simulink model "time_gongji_KVHonline"  (R2019b)
settings: Solver=ode3  StartTime=0.0  StopTime=6000  FixedStep=0.01  MaxStep=0.01  RelTol=1e-3
values from neighbouring files (symbols this model uses):
  bias_gyro_z_gongji = 2e-3    (= 0.002)    [sych_ite_KVHonline_daoyuan_huace.m]
settings Model: Creator=luyishi_E480  LastModifiedBy=xie_z
settings DataIOCC: SaveOutput=off  SignalLogging=off  DSMLogging=off  InspectSignalLogs=on  SaveTime=off  ReturnWorkspaceOutputs=off
settings DebuggingCC: InheritedTsInSrcMsg=none

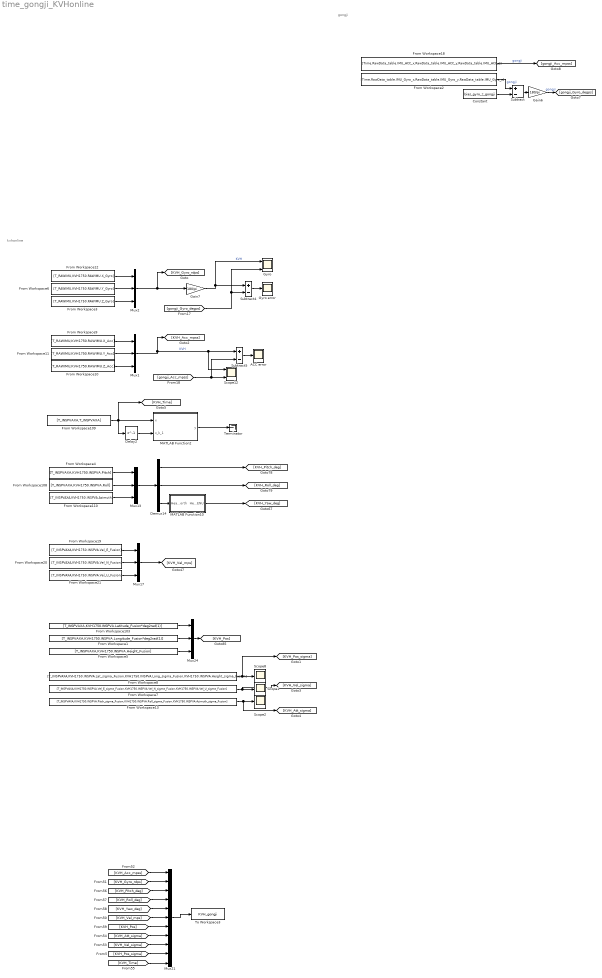
== system time_gongji_KVHonline ==
  note: gongji
  note: kvhonline
  ACC error : Scope
  Constant : Constant  Value=bias_gyro_z_gongji
  Delay2 : Delay  DelayLength=1  InitialCondition=0
  Demux14 : Demux  Outputs=3
  From Workspace1 : FromWorkspace  VariableName=[T_INSPVAXA,KVH1750.INSPVA.Longitude_Fusion*deg2rad(1)]  OutputAfterFinalValue=Holding final value
  From Workspace10 : FromWorkspace  VariableName=[T_RAWIMU,KVH1750.RAWIMU.Z_Acc]  Interpolate=off  OutputAfterFinalValue=Holding final value
  From Workspace103 : FromWorkspace  VariableName=[T_INSPVAXA,KVH1750.INSPVA.Latitude_Fusion*deg2rad(1)]  OutputAfterFinalValue=Holding final value
  From Workspace108 : FromWorkspace  VariableName=[T_INSPVAXA,KVH1750.INSPVA.Roll]  Interpolate=off  OutputAfterFinalValue=Holding final value
  From Workspace109 : FromWorkspace  VariableName=[T_INSPVAXA,T_INSPVAXA]  Interpolate=off  OutputAfterFinalValue=Holding final value
  From Workspace11 : FromWorkspace  VariableName=[T_RAWIMU,KVH1750.RAWIMU.Y_Acc]  Interpolate=off  OutputAfterFinalValue=Holding final value
  From Workspace110 : FromWorkspace  VariableName=[T_INSPVAXA,KVH1750.INSPVA.Azimuth]  Interpolate=off  OutputAfterFinalValue=Holding final value
  From Workspace12 : FromWorkspace  VariableName=[T_RAWIMU,KVH1750.RAWIMU.X_Gyro]  Interpolate=off  OutputAfterFinalValue=Holding final value
  From Workspace13 : FromWorkspace  VariableName=[T_INSPVAXA,KVH1750.INSPVA.Pitch_sigma_Fusion,KVH1750.INSPVA.Roll_sigma_Fusion,KVH1750.INSPVA.Azimuth_sigma_Fusion]  Interpolate=off  OutputAfterFinalValue=Holding final value
  From Workspace18 : FromWorkspace  VariableName=[Time,RawData_table.IMU_ACC_x,RawData_table.IMU_ACC_y,RawData_table.IMU_ACC_z]  Interpolate=off  OutputAfterFinalValue=Holding final value
  From Workspace19 : FromWorkspace  VariableName=[T_INSPVAXA,KVH1750.INSPVA.Vel_E_Fusion]  Interpolate=off  OutputAfterFinalValue=Holding final value
  From Workspace2 : FromWorkspace  VariableName=[Time,RawData_table.IMU_Gyro_x,RawData_table.IMU_Gyro_y,RawData_table.IMU_Gyro_z]  Interpolate=off  OutputAfterFinalValue=Holding final value
  From Workspace20 : FromWorkspace  VariableName=[T_INSPVAXA,KVH1750.INSPVA.Vel_N_Fusion]  Interpolate=off  OutputAfterFinalValue=Holding final value
  From Workspace21 : FromWorkspace  VariableName=[T_INSPVAXA,KVH1750.INSPVA.Vel_U_Fusion]  Interpolate=off  OutputAfterFinalValue=Holding final value
  From Workspace3 : FromWorkspace  VariableName=[T_RAWIMU,KVH1750.RAWIMU.Z_Gyro]  Interpolate=off  OutputAfterFinalValue=Holding final value
  From Workspace4 : FromWorkspace  VariableName=[T_INSPVAXA,KVH1750.INSPVA.Pitch]  Interpolate=off  OutputAfterFinalValue=Holding final value
  From Workspace5 : FromWorkspace  VariableName=[T_INSPVAXA,KVH1750.INSPVA.Height_Fusion]  OutputAfterFinalValue=Holding final value
  From Workspace6 : FromWorkspace  VariableName=[T_RAWIMU,KVH1750.RAWIMU.Y_Gyro]  Interpolate=off  OutputAfterFinalValue=Holding final value
  From Workspace7 : FromWorkspace  VariableName=[T_INSPVAXA,KVH1750.INSPVA.Vel_E_sigma_Fusion,KVH1750.INSPVA.Vel_N_sigma_Fusion,KVH1750.INSPVA.Vel_U_sigma_Fusion]  Interpolate=off  OutputAfterFinalValue=Holding final value
  From Workspace8 : FromWorkspace  VariableName=[T_INSPVAXA,KVH1750.INSPVA.Lat_sigma_Fusion,KVH1750.INSPVA.Long_sigma_Fusion,KVH1750.INSPVA.Height_sigma_Fusion]  Interpolate=off  OutputAfterFinalValue=Holding final value
  From Workspace9 : FromWorkspace  VariableName=[T_RAWIMU,KVH1750.RAWIMU.X_Acc]  Interpolate=off  OutputAfterFinalValue=Holding final value
  Gain6 : Gain  Gain=180/pi
  Gain7 : Gain  Gain=180/pi
  "Gyro " : Scope  NumInputPorts=2
  Gyro error : Scope
  MATLAB Function10 : MATLAB Function  TreatAsAtomicUnit=on
  MATLAB Function2 : MATLAB Function  TreatAsAtomicUnit=on
  Mux{1..2,13,17,24} (5 alike) : Mux  Inputs=3
  Mux21 : Mux  Inputs=11
  Scope1 : Scope
  Scope12 : Scope  NumInputPorts=2
  Scope2 : Scope
  Scope8 : Scope
  Subtract : Sum  Inputs=+-
  Subtract4 : Sum  Inputs=+-
  Subtract5 : Sum  Inputs=+-
  Terminator : Terminator
  To Workspace3 : ToWorkspace  VariableName=KVH_gongji  SaveFormat=Structure With Time  SampleTime=-1
  wires:
  Mux2/1 -> [KVH_Gyro_rdps], Gain7/1
  Subtract4/1 -> Gyro error/1
  Subtract5/1 -> ACC error/1
  Gain7/1 -> "Gyro "/1, Subtract4/1  "KVH"
  Mux1/1 -> [KVH_Acc_mpss], Subtract5/1, Scope12/1  "KVH"
  From Workspace9/1 -> Mux1/1
  From Workspace11/1 -> Mux1/2
  From Workspace10/1 -> Mux1/3
  From Workspace3/1 -> Mux2/3
  From Workspace6/1 -> Mux2/2
  From Workspace12/1 -> Mux2/1
  Subtract/1 -> Gain6/1
  Constant/1 -> Subtract/2
  From Workspace2/1 -> Subtract/1  "gongji"
  From Workspace18/1 -> [gongji_Acc_mpss]  "gongji"
  Gain6/1 -> [gongji_Gyro_degps]  "gongji"
  [gongji_Gyro_degps] -> Subtract4/2, "Gyro "/2
  [gongji_Acc_mpss] -> Subtract5/2, Scope12/2
  MATLAB Function2/1(y) -> Terminator/1
  Delay2/1 -> MATLAB Function2/2(x_k_1)
  From Workspace109/1 -> [KVH_Time], Delay2/1, MATLAB Function2/1(x)
  Demux14/1 -> [KVH_Pitch_deg]
  From Workspace4/1 -> Mux13/1
  Demux14/3 -> MATLAB Function10/1(Heading_North)
  Demux14/2 -> [KVH_Roll_deg]
  From Workspace110/1 -> Mux13/3
  From Workspace108/1 -> Mux13/2
  Mux13/1 -> Demux14/1
  MATLAB Function10/1(Heading_ENU) -> [KVH_Yaw_deg]
  From Workspace21/1 -> Mux17/3
  From Workspace19/1 -> Mux17/1
  From Workspace20/1 -> Mux17/2
  Mux17/1 -> [KVH_Vel_mps]
  From Workspace5/1 -> Mux24/3
  From Workspace7/1 -> [KVH_Vel_sigma], Scope1/1
  From Workspace13/1 -> [KVH_Att_sigma], Scope2/1
  Mux24/1 -> [KVH_Pos]
  From Workspace103/1 -> Mux24/1
  From Workspace1/1 -> Mux24/2
  From Workspace8/1 -> [KVH_Pos_sigma], Scope8/1
  [KVH_Pos_sigma] -> Mux21/10
  [KVH_Att_sigma] -> Mux21/8
  [KVH_Acc_mpss] -> Mux21/1
  Mux21/1 -> To Workspace3/1
  [KVH_Pitch_deg] -> Mux21/3
  [KVH_Time] -> Mux21/11
  [KVH_Vel_mps] -> Mux21/6
  [KVH_Yaw_deg] -> Mux21/5
  [KVH_Roll_deg] -> Mux21/4
  [KVH_Pos] -> Mux21/7
  [KVH_Gyro_rdps] -> Mux21/2
  [KVH_Vel_sigma] -> Mux21/9

== matlab function time_gongji_KVHonline/MATLAB Function2 ==
  data: y output; x input; x_k_1 input
function y  = fcn(x,x_k_1)
    if x ~= x_k_1
        y = uint8(1);
    else
        y = uint8(0);
    end
end

== matlab function time_gongji_KVHonline/MATLAB Function10 ==
  data: Heading_North input; Heading_ENU output size=1
function Heading_ENU = fcn(Heading_North)
% Heading_ENU:以北为零顺时针为正0-360°
% Heading_North:以北为零逆时针为正-180-180°

% Heading_North = Heading_North + 0.5 + 3.8;
if Heading_North <= 180
    Heading_ENU = 0 - Heading_North;
else
    Heading_ENU = 360 - Heading_North;
end
